simulink model "avion_fstd"  (R2021b)
settings: Solver=ode45  StartTime=0.0  StopTime=10.0  RelTol=1e-3  EnableMultiTasking=on
values from neighbouring files (symbols this model uses):
  a = [ -0.1400    0.0530   -0.9990    0.0470 ... (first row only)    [demarrage.m]
  b = [0 0.03;0.404   0.26;0.00  -0.68;0 0]    [demarrage.m]
  c = [ 0.0433   -0.0003    0.0016         0;          0    1.0000         0      0;          0         0    1.0000      0 ;          0         0         0    1.0000]    [demarrage.m]
  d = [0.0001   -0.0075;0 0;0 0;0 0]    [demarrage.m]
libraries: cstblocks x2
settings Model: Creator=d.alazard  LastModifiedBy=driss
settings SolverCC: AlgebraicLoopSolver=TrustRegion
settings DataIOCC: LimitDataPoints=on  SaveFormat=Array  SignalLoggingSaveFormat=ModelDataLogs  ReturnWorkspaceOutputs=off
settings OptimizationCC: BlockReduction=off  BooleanDataType=off  ExpressionDepthLimit=2147483647  LifeSpan=inf
settings DebuggingCC: SaveWithParameterizedLinksMsg=none  UnderspecifiedInitializationDetection=Classic  MergeDetectMultiDrivingBlocksExec=none  SignalResolutionControl=TryResolveAllWithWarning  MultiTaskDSMMsg=warning  MultiTaskCondExecSysMsg=none  FcnCallInpInsideContextMsg=warning  StateNameClashWarn=warning  SFUnexpectedBacktrackingDiag=warning  SFNoUnconditionalDefaultTransitionDiag=warning  SFExecutionAtInitializationDiag=none  SFMachineParentedDataDiag=warning  ArithmeticOperatorsInVariantConditions=warning
settings HardwareCC: ProdBitPerPointer=32  ProdBitPerSizeT=32  ProdBitPerPtrDiffT=32  ProdLargestAtomicFloat=None  ProdIntDivRoundTo=Undefined  ProdEndianess=Unspecified  ProdWordSize=32  ProdHWDeviceType=32-bit Generic  TargetUnknown=on
settings ModelReferenceCC: PropagateSignalLabelsOutOfModel=off
settings SFSimCC: SimUseLocalCustomCode=off  CustomCodeUndefinedFunction=UseInterfaceOnly
settings RTWCC: RTWUseLocalCustomCode=off
settings CodeAppCC: StateflowObjectComments=on
settings GRTTargetCC: TargetLangStandard=C89/C90 (ANSI)  CombineOutputUpdateFcns=off  GRTInterface=on
settings ConfigComp: CovMetricSettings=dw  CovSaveCumulativeToWorkspaceVar=on  CovSaveSingleToWorkspaceVar=on  CovExternalEMLEnable=off

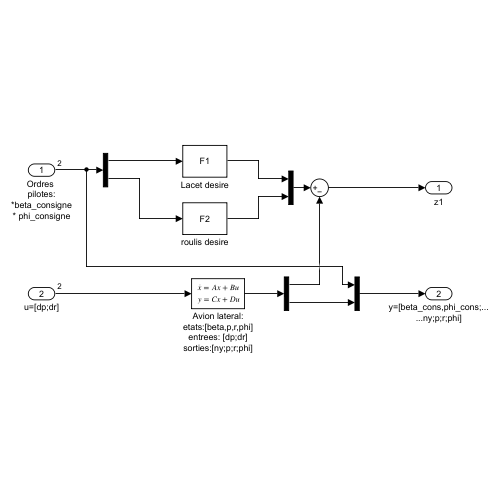
[thumbnail: Simulink's stored preview of the top-level diagram]
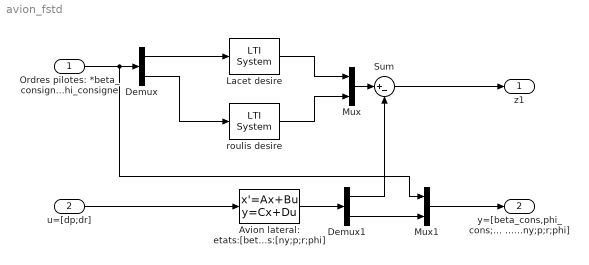
== system avion_fstd ==
  Ordres pilotes: *beta_consigne * phi_consigne : Inport  PortDimensions=2
  u=[dp;dr] : Inport  Port=2  PortDimensions=2
  Avion lateral: etats:[beta,p,r,phi] entrees: [dp;dr] sorties:[ny;p;r;phi] : StateSpace  A=a  B=b  C=[1 0 0 0;0 0 0 1;c]  D=[0 0;0 0;d]  InitialCondition=0
  Demux : Demux  Outputs=2
      settings: DisplayOption=none
  Demux1 : Demux  Outputs=[2 4]
      settings: DisplayOption=none
  Lacet desire : cstblocks/LTI System  sys=F1  IC=[]
  Mux : Mux  Inputs=2
  Mux1 : Mux  Inputs=[2 4]
  Sum : Sum  Inputs=|+-  InputSameDT=on  SaturateOnIntegerOverflow=on  OutDataTypeStr=Inherit: Same as first input
  roulis desire : cstblocks/LTI System  sys=F2  IC=[]
  z1 : Outport  VectorParamsAs1DForOutWhenUnconnected=off
  y=[beta_cons,phi_cons;... ...ny;p;r;phi] : Outport  Port=2  VectorParamsAs1DForOutWhenUnconnected=off
  wires:
  Ordres pilotes: *beta_consigne * phi_consigne/1 -> Demux/1, Mux1/1
  Demux/1 -> Lacet desire/1
  Demux/2 -> roulis desire/1
  Lacet desire/1 -> Mux/1
  roulis desire/1 -> Mux/2
  Avion lateral: etats:[beta,p,r,phi] entrees: [dp;dr] sorties:[ny;p;r;phi]/1 -> Demux1/1
  Demux1/1 -> Sum/2
  Mux/1 -> Sum/1
  Sum/1 -> z1/1
  Demux1/2 -> Mux1/2
  Mux1/1 -> y=[beta_cons,phi_cons;... ...ny;p;r;phi]/1
  u=[dp;dr]/1 -> Avion lateral: etats:[beta,p,r,phi] entrees: [dp;dr] sorties:[ny;p;r;phi]/1
